simulink model "FourToOneMultiplexor"  (R2017b)
settings: Solver=VariableStepAuto  StartTime=0.0  StopTime=10.0  RelTol=1e-3
settings Model: Creator=Ray  LastModifiedBy=Ray

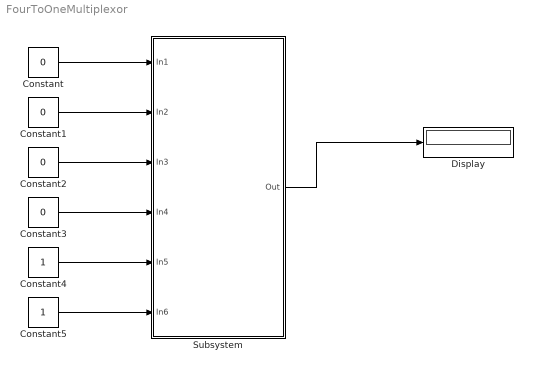
== system FourToOneMultiplexor ==
  Constant{,1..3} (4 alike) : Constant  Value=0  OutDataTypeStr=boolean  SampleTime=1
  Constant4 : Constant  OutDataTypeStr=boolean  SampleTime=1
  Constant5 : Constant  OutDataTypeStr=boolean  SampleTime=1
  Display : Display
  Subsystem : Subsystem
  wires:
  Subsystem/1(Out) -> Display/1
  Constant/1 -> Subsystem/1(In1)
  Constant1/1 -> Subsystem/2(In2)
  Constant2/1 -> Subsystem/3(In3)
  Constant3/1 -> Subsystem/4(In4)
  Constant4/1 -> Subsystem/5(In5)
  Constant5/1 -> Subsystem/6(In6)

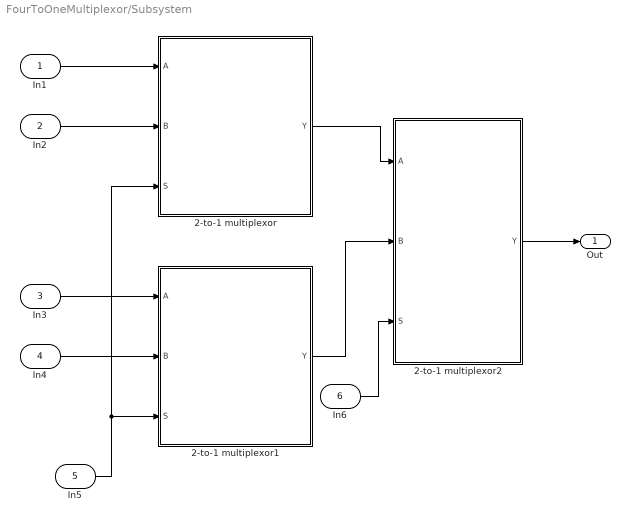
== system FourToOneMultiplexor/Subsystem ==
  In1 : Inport  OutDataTypeStr=boolean  SampleTime=1
  In2 : Inport  Port=2  OutDataTypeStr=boolean  SampleTime=1
  In3 : Inport  Port=3  OutDataTypeStr=boolean  SampleTime=1
  In4 : Inport  Port=4  OutDataTypeStr=boolean  SampleTime=1
  In5 : Inport  Port=5  OutDataTypeStr=boolean  SampleTime=1
  In6 : Inport  Port=6  OutDataTypeStr=boolean  SampleTime=1
  2-to-1 multiplexor : Subsystem
  2-to-1 multiplexor1 : Subsystem
  2-to-1 multiplexor2 : Subsystem
  Out : Outport
  wires:
  In6/1 -> 2-to-1 multiplexor2/3(S)
  2-to-1 multiplexor2/1(Y) -> Out/1
  In5/1 -> 2-to-1 multiplexor/3(S), 2-to-1 multiplexor1/3(S)
  In4/1 -> 2-to-1 multiplexor1/2(B)
  2-to-1 multiplexor1/1(Y) -> 2-to-1 multiplexor2/2(B)
  2-to-1 multiplexor/1(Y) -> 2-to-1 multiplexor2/1(A)
  In2/1 -> 2-to-1 multiplexor/2(B)
  In1/1 -> 2-to-1 multiplexor/1(A)
  In3/1 -> 2-to-1 multiplexor1/1(A)

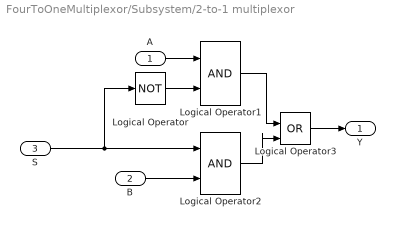
== system FourToOneMultiplexor/Subsystem/2-to-1 multiplexor ==
  A : Inport  OutDataTypeStr=boolean  SampleTime=1
  B : Inport  Port=2  OutDataTypeStr=boolean  SampleTime=1
  S : Inport  Port=3  OutDataTypeStr=boolean  SampleTime=1
  Logical Operator : Logic  Operator=NOT  IconShape=distinctive  AllPortsSameDT=off  OutDataTypeStr=boolean
  Logical Operator1 : Logic  IconShape=distinctive  AllPortsSameDT=off  OutDataTypeStr=boolean
  Logical Operator2 : Logic  IconShape=distinctive  AllPortsSameDT=off  OutDataTypeStr=boolean
  Logical Operator3 : Logic  Operator=OR  IconShape=distinctive  AllPortsSameDT=off  OutDataTypeStr=boolean
  Y : Outport
  wires:
  Logical Operator2/1 -> Logical Operator3/2
  Logical Operator1/1 -> Logical Operator3/1
  Logical Operator3/1 -> Y/1
  A/1 -> Logical Operator1/1
  S/1 -> Logical Operator2/1, Logical Operator/1
  B/1 -> Logical Operator2/2
  Logical Operator/1 -> Logical Operator1/2

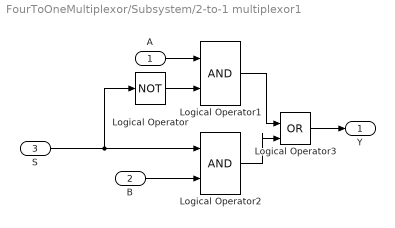
== system FourToOneMultiplexor/Subsystem/2-to-1 multiplexor1 ==
  A : Inport  OutDataTypeStr=boolean  SampleTime=1
  B : Inport  Port=2  OutDataTypeStr=boolean  SampleTime=1
  S : Inport  Port=3  OutDataTypeStr=boolean  SampleTime=1
  Logical Operator : Logic  Operator=NOT  IconShape=distinctive  AllPortsSameDT=off  OutDataTypeStr=boolean
  Logical Operator1 : Logic  IconShape=distinctive  AllPortsSameDT=off  OutDataTypeStr=boolean
  Logical Operator2 : Logic  IconShape=distinctive  AllPortsSameDT=off  OutDataTypeStr=boolean
  Logical Operator3 : Logic  Operator=OR  IconShape=distinctive  AllPortsSameDT=off  OutDataTypeStr=boolean
  Y : Outport
  wires:
  Logical Operator2/1 -> Logical Operator3/2
  Logical Operator1/1 -> Logical Operator3/1
  Logical Operator3/1 -> Y/1
  A/1 -> Logical Operator1/1
  S/1 -> Logical Operator2/1, Logical Operator/1
  B/1 -> Logical Operator2/2
  Logical Operator/1 -> Logical Operator1/2

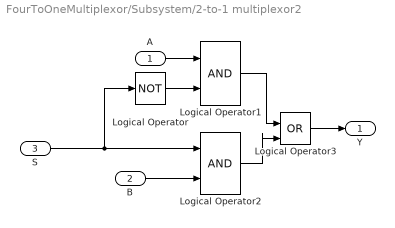
== system FourToOneMultiplexor/Subsystem/2-to-1 multiplexor2 ==
  A : Inport  OutDataTypeStr=boolean  SampleTime=1
  B : Inport  Port=2  OutDataTypeStr=boolean  SampleTime=1
  S : Inport  Port=3  OutDataTypeStr=boolean  SampleTime=1
  Logical Operator : Logic  Operator=NOT  IconShape=distinctive  AllPortsSameDT=off  OutDataTypeStr=boolean
  Logical Operator1 : Logic  IconShape=distinctive  AllPortsSameDT=off  OutDataTypeStr=boolean
  Logical Operator2 : Logic  IconShape=distinctive  AllPortsSameDT=off  OutDataTypeStr=boolean
  Logical Operator3 : Logic  Operator=OR  IconShape=distinctive  AllPortsSameDT=off  OutDataTypeStr=boolean
  Y : Outport
  wires:
  Logical Operator2/1 -> Logical Operator3/2
  Logical Operator1/1 -> Logical Operator3/1
  Logical Operator3/1 -> Y/1
  A/1 -> Logical Operator1/1
  S/1 -> Logical Operator2/1, Logical Operator/1
  B/1 -> Logical Operator2/2
  Logical Operator/1 -> Logical Operator1/2
